simulink model "suspm"  (R2023b)
settings: Solver=VariableStepAuto  StartTime=0.0  StopTime=10.0  RelTol=1e-3
values from neighbouring files (symbols this model uses):
  b1 = 1000    [parameters_suspension.m]
  b2 = 150000    [parameters_suspension.m]
  k1 = 30000    [parameters_suspension.m]
  k2 = 100000    [parameters_suspension.m]
  m1 = 1000    [parameters_suspension.m]
  m2 = 20    [parameters_suspension.m]
settings Model: Creator=martinhaugen  LastModifiedBy=martinhaugen

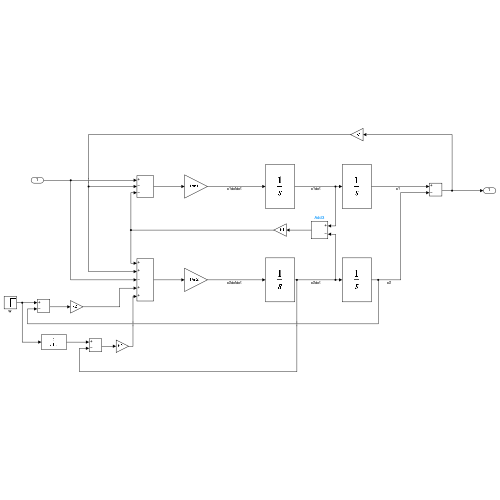
[thumbnail: Simulink's stored preview of the top-level diagram]
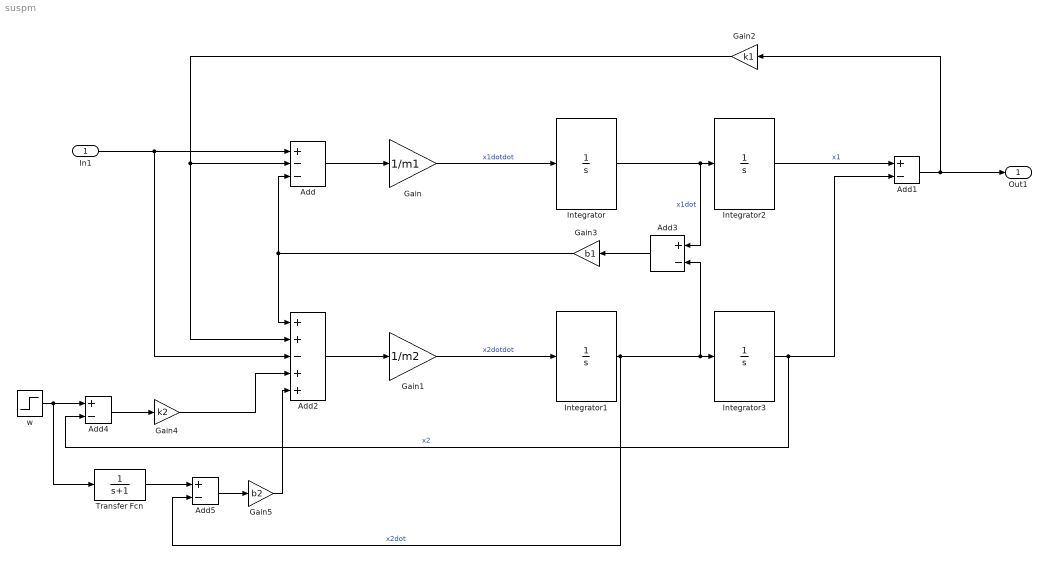
== system suspm ==
  In1 : Inport
  Add : Sum  Inputs=+--
  Add{1,3..5} (4 alike) : Sum  Inputs=+-
  Add2 : Sum  Inputs=++-++
  Gain : Gain  Gain=1/m1
  Gain1 : Gain  Gain=1/m2
  Gain2 : Gain  Gain=k1
  Gain3 : Gain  Gain=b1
  Gain4 : Gain  Gain=k2
  Gain5 : Gain  Gain=b2
  Integrator{,1..3} (4 alike) : Integrator
  Transfer Fcn : TransferFcn  Denominator=[1 1]
  w : Step  After=0  SampleTime=0
  Out1 : Outport
  wires:
  Integrator/1 -> Add3/1, Integrator2/1  "x1dot"
  Integrator2/1 -> Add1/1  "x1"
  Gain/1 -> Integrator/1  "x1dotdot"
  Gain1/1 -> Integrator1/1  "x2dotdot"
  Integrator1/1 -> Add5/2, Integrator3/1, Add3/2  "x2dot"
  Integrator3/1 -> Add4/2, Add1/2  "x2"
  Add/1 -> Gain/1
  Add1/1 -> Out1/1, Gain2/1
  Gain2/1 -> Add2/2, Add/2
  Add2/1 -> Gain1/1
  Add3/1 -> Gain3/1
  Gain3/1 -> Add2/1, Add/3
  In1/1 -> Add/1, Add2/3
  w/1 -> Transfer Fcn/1, Add4/1
  Gain4/1 -> Add2/4
  Add4/1 -> Gain4/1
  Transfer Fcn/1 -> Add5/1
  Add5/1 -> Gain5/1
  Gain5/1 -> Add2/5
